simulink model "UAM_controller"  (R2024b)
settings: Solver=VariableStepAuto  StartTime=0.0  StopTime=10.0  RelTol=1e-3
settings Model: Creator=admin  LastModifiedBy=admin

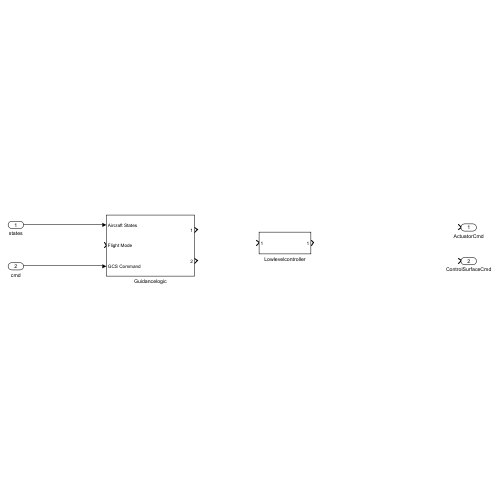
[thumbnail: Simulink's stored preview of the top-level diagram]
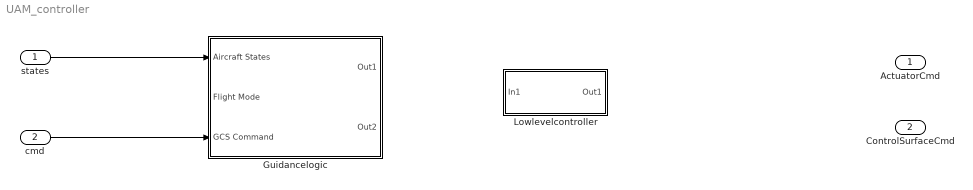
== system UAM_controller ==
  states : Inport
  cmd : Inport  Port=2
  Guidancelogic : Subsystem
  Lowlevelcontroller : Subsystem
  ActuatorCmd : Outport
  ControlSurfaceCmd : Outport  Port=2
  wires:
  states/1 -> Guidancelogic/1(Aircraft States)
  cmd/1 -> Guidancelogic/3(GCS Command)

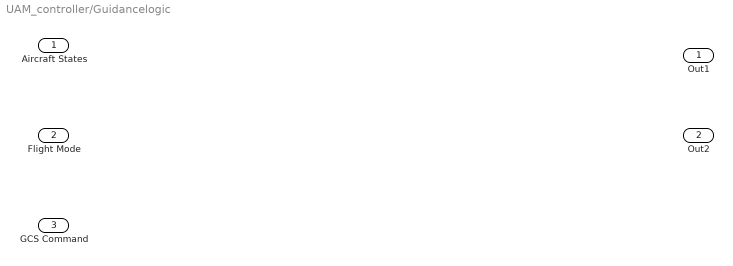
== system UAM_controller/Guidancelogic ==
  Aircraft States : Inport
  Flight Mode : Inport  Port=2
  GCS Command : Inport  Port=3
  Out1 : Outport
  Out2 : Outport  Port=2

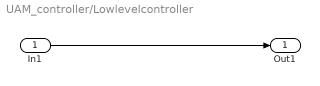
== system UAM_controller/Lowlevelcontroller ==
  In1 : Inport
  Out1 : Outport
  wires:
  In1/1 -> Out1/1
